simulink library "uavsimBlockset_LateralEulerAttitudeController"  (Simulink 8.0)
settings: Solver=ode45  StartTime=0.0  StopTime=10.0  RelTol=1e-3
undefined symbols (not defined in the file): aircraftLibraryData, DiscIntNeverNeededParam
settings Model: Creator=mstolle  LastModifiedBy=j.bolting

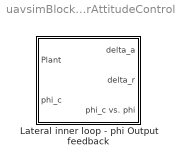
== system uavsimBlockset_LateralEulerAttitudeController ==
  Lateral inner loop - phi Output feedback : Subsystem  mask{mask_K=aircraftLibraryData.zagi.control.gains.Klateral_phi}
      mask prompts: mask_K "Feedback gain matrix K"

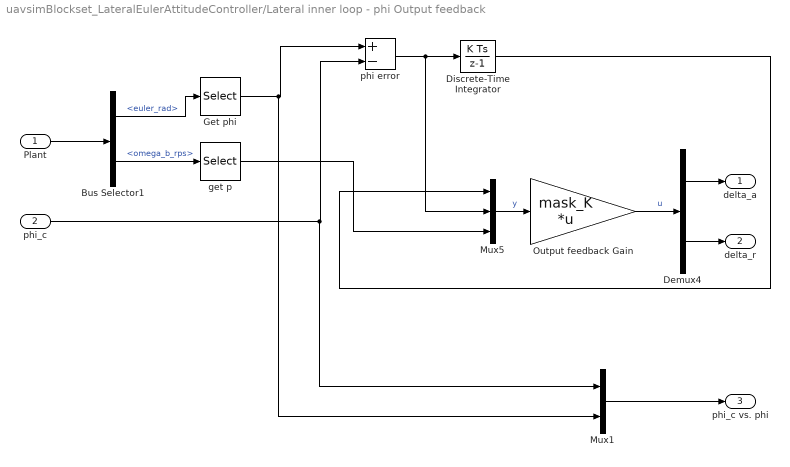
== system uavsimBlockset_LateralEulerAttitudeController/Lateral inner loop - phi Output feedback ==
  Plant : Inport  OutDataTypeStr=Bus: Airframe
  phi_c : Inport  Port=2
  Bus Selector1 : BusSelector  OutputSignals=Kinematics.Attitude.euler_rad,Kinematics.RotationalVelocity.omega_b_rps
  Demux4 : Demux  Outputs=2
  Discrete-Time Integrator : DiscreteIntegrator  SampleTime=-1  ICPrevOutput=DiscIntNeverNeededParam  ICPrevScaledInput=DiscIntNeverNeededParam
  Get phi : Selector  InputPortWidth=3  IndexOptions=Index vector (dialog)  Indices=1  OutputSizes=1
  Mux1 : Mux  Inputs=2
  Mux5 : Mux  Inputs=3
  Output feedback Gain : Gain  Gain=mask_K  Multiplication=Matrix(K*u)
  get p : Selector  InputPortWidth=3  IndexOptions=Index vector (dialog)  Indices=1  OutputSizes=1
  phi error : Sum  Inputs=+-
  delta_a : Outport
  delta_r : Outport  Port=2
  phi_c vs. phi : Outport  Port=3
  wires:
  phi error/1 -> Mux5/2, Discrete-Time Integrator/1
  Discrete-Time Integrator/1 -> Mux5/1
  Demux4/2 -> delta_r/1
  Demux4/1 -> delta_a/1
  Output feedback Gain/1 -> Demux4/1  "u"
  Mux5/1 -> Output feedback Gain/1  "y"
  phi_c/1 -> Mux1/1, phi error/2
  Plant/1 -> Bus Selector1/1
  Bus Selector1/2 -> get p/1  "<omega_b_rps>"
  Bus Selector1/1 -> Get phi/1  "<euler_rad>"
  Get phi/1 -> Mux1/2, phi error/1
  get p/1 -> Mux5/3
  Mux1/1 -> phi_c vs. phi/1
